simulink model "LQ_integrator_pendulum_anim"  (R2016b)
settings: Solver=ode45  StartTime=0.0  StopTime=inf  RelTol=1e-3  EnableMultiTasking=on
values from neighbouring files (symbols this model uses):
  g = 9.81    [pendulum_sys_init_solution.m]
  K_LQ = lqr(A_int,B_int,Q,R)    [pendulum_sys_init_solution.m]
  kc = 2    [pendulum_sys_init_solution.m]
  ke = 2    [pendulum_sys_init_solution.m]
  l = 1    [pendulum_sys_init_solution.m]
  M = 10    [pendulum_sys_init_solution.m]
  m = 2    [pendulum_sys_init_solution.m]
  ra = 10    [pendulum_sys_init_solution.m]
  rr = .1    (= 0.1)    [pendulum_sys_init_solution.m]
undefined symbols (not defined in the file or in its folder): pendolo_sys_diff
libraries: simulink x1, vrlib x1
settings Model: Creator=Titano  LastModifiedBy=AlessioLaBella
settings DataIOCC: LimitDataPoints=on  SaveFormat=Array  SignalLoggingSaveFormat=ModelDataLogs
settings OptimizationCC: ExpressionDepthLimit=2147483647  InitFltsAndDblsToZero=on  LifeSpan=inf
settings DebuggingCC: UnderspecifiedInitializationDetection=Classic  MergeDetectMultiDrivingBlocksExec=none  SolverPrmCheckMsg=warning  FcnCallInpInsideContextMsg=warning  StateNameClashWarn=warning  SFUnexpectedBacktrackingDiag=warning  SFNoUnconditionalDefaultTransitionDiag=warning  SFExecutionAtInitializationDiag=none
settings HardwareCC: ProdBitPerPointer=32  ProdBitPerSizeT=32  ProdBitPerPtrDiffT=32  ProdLargestAtomicFloat=None  ProdIntDivRoundTo=Undefined  ProdEndianess=Unspecified  ProdWordSize=32  ProdHWDeviceType=32-bit Generic
settings ModelReferenceCC: PropagateSignalLabelsOutOfModel=off
settings GRTTargetCC: TargetLangStandard=C89/C90 (ANSI)  GeneratePreprocessorConditionals=Disable all  CombineOutputUpdateFcns=off  GRTInterface=on
settings ConfigComp: CovMetricSettings=dw  CovHtmlReporting=on  CovSaveCumulativeToWorkspaceVar=on  CovSaveSingleToWorkspaceVar=on  CovExternalEMLEnable=off
settings SimMechanicsCC: VisDuringSimulation=on
settings ConfigurationSet: Description=SimMechanics 2G

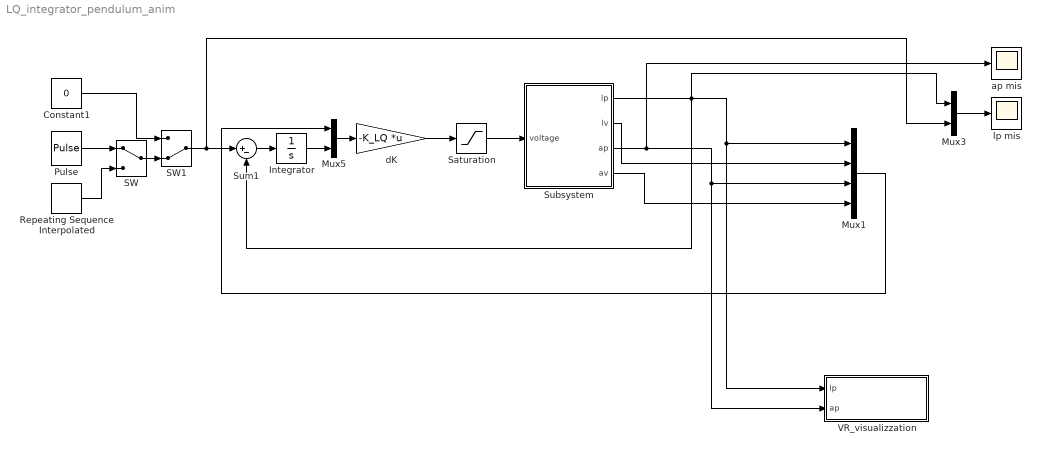
== system LQ_integrator_pendulum_anim ==
  Constant1 : Constant  Value=0
  Integrator : Integrator
  Mux1 : Mux
  Mux3 : Mux  Inputs=2
  Mux5 : Mux  Inputs=2
  Pulse : DiscretePulseGenerator  PulseType=Time based  Amplitude=.5  Period=20  PulseWidth=50
  Repeating Sequence Interpolated : simulink/Sources/Repeating Sequence Interpolated  OutValues=[.5 -.5 -.5 .5 .5].'  TimeValues=[0 2.5 5 7.5 10].'  LookUpMeth=Interpolation-Use End Values  tsamp=0.01  OutMin=[]  OutMax=[]  OutDataTypeStr=float('double')  OutputDataTypeScalingMode=Specify via dialog  OutDataType=float('double')  OutScaling=2^-10
  SW : ManualSwitch
  SW1 : ManualSwitch  CurrentSetting=0
  Saturation : Saturate  UpperLimit=24  LowerLimit=-24
  Subsystem : Subsystem
  Sum1 : Sum  Inputs=|+-
  VR_visualizzation : Subsystem
  ap mis : Scope
  dK : Gain  Gain=-K_LQ  Multiplication=Matrix(K*u)
  lp mis : Scope
  wires:
  Subsystem/3(ap) -> ap mis/1, Mux1/3, VR_visualizzation/2(ap)
  Subsystem/1(lp) -> Mux3/1, Sum1/2, VR_visualizzation/1(lp), Mux1/1
  Mux3/1 -> lp mis/1
  Constant1/1 -> SW1/1
  Mux1/1 -> Mux5/1
  SW1/1 -> Mux3/2, Sum1/1
  Sum1/1 -> Integrator/1
  Integrator/1 -> Mux5/2
  Mux5/1 -> dK/1
  SW/1 -> SW1/2
  Pulse/1 -> SW/1
  Repeating Sequence Interpolated/1 -> SW/2
  Subsystem/2(lv) -> Mux1/2
  Subsystem/4(av) -> Mux1/4
  dK/1 -> Saturation/1
  Saturation/1 -> Subsystem/1(voltage)

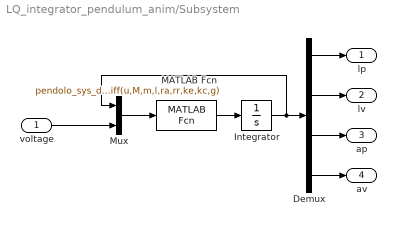
== system LQ_integrator_pendulum_anim/Subsystem ==
  voltage : Inport
  Demux : Demux
  Integrator : Integrator  InitialCondition=[0 0 0.1 0]
  MATLAB Fcn : MATLABFcn  MATLABFcn=pendolo_sys_diff(u,M,m,l,ra,rr,ke,kc,g)
  Mux : Mux  Inputs=2
  lp : Outport
  lv : Outport  Port=2
  ap : Outport  Port=3
  av : Outport  Port=4
  wires:
  MATLAB Fcn/1 -> Integrator/1
  Integrator/1 -> Demux/1, Mux/1
  Demux/4 -> av/1
  Demux/3 -> ap/1
  Demux/2 -> lv/1
  Demux/1 -> lp/1
  Mux/1 -> MATLAB Fcn/1
  voltage/1 -> Mux/2

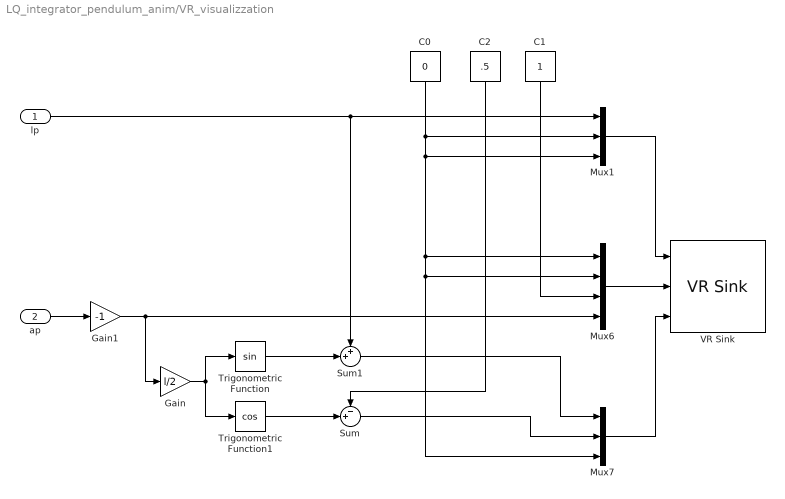
== system LQ_integrator_pendulum_anim/VR_visualizzation ==
  lp : Inport
  ap : Inport  Port=2
  C0 : Constant  Value=0
  C1 : Constant
  C2 : Constant  Value=.5
  Gain : Gain  Gain=l/2
  Gain1 : Gain  Gain=-1
  Mux1 : Mux  Inputs=3
  Mux6 : Mux
  Mux7 : Mux  Inputs=3
  Sum : Sum  Inputs=-+|
  Sum1 : Sum  Inputs=++|
  Trigonometric Function : Trigonometry
  Trigonometric Function1 : Trigonometry  Operator=cos
  VR Sink : vrlib/VR Sink  InstantiateOnLoad=on  SampleTime=0.02  ViewEnable=on  RemoteChange=off  RemoteView=off  FieldsWritten=carrello.translation.3.1.double#asta.rotation.4.1.double#asta.translation.3.1.double  WorldFileName=vrml1.wrl  AutoView=on  VideoDimensions=[]  AllowVariableSize=off  FigureProperties="{'Position', 'Name', 'Viewpoint', 'CameraBound', 'CameraDirection', 'CameraPosition', 'CameraUpVector', 'ZoomFactor', 'Antialiasing', 'Headlight', 'Lighting', 'NavPanel', 'Sound', 'StatusBar', 'Stereo3D', 'Stereo3DCameraOffset', 'Stereo3DHIT', 'ToolBar', 'Textures', 'Transparency', 'Triad', 'Wireframe', 'NavZones', 'NavMode', 'NavSpeed', 'CaptureFileFormat', 'CaptureFileName', 'Record2DCompressMethod', 'Record2DCompressQuality', 'Record2D', 'Record2DFileName', 'Record2DFPS'; [5.0000000000000000e+00   9.2333333333333371e+01   5.7600000000000000e+02   3.5000000000000000e+02], '', '', 'on', [0.0000000000000000e+00   0.0000000000000000e+00  -1.0000000000000000e+00], [0.0000000000000000e+00   0.0000000000000000e+00   1.0000000000000000e+01], [0.0000000000000000e+00   1.0000000000000000e+00   0.0000000000000000e+00], [1.0000000000000000e+00], 'on', 'on', 'on', 'halfbar', 'on', 'on', 'off', [1.0000000149011612e-01], [0.0000000000000000e+00], 'on', 'on', 'on', 'none', 'off', 'off', 'walk', 'normal', 'tif', '%f_anim_%n.tif', 'auto', [7.5000000000000000e+01], 'off', '%f_anim_%n.avi', 'auto'}"
  wires:
  Mux1/1 -> VR Sink/1
  Mux6/1 -> VR Sink/2
  Mux7/1 -> VR Sink/3
  lp/1 -> Mux1/1, Sum1/1
  C0/1 -> Mux1/2, Mux1/3, Mux6/1, Mux6/2, Mux7/3
  ap/1 -> Gain1/1
  C1/1 -> Mux6/3
  Trigonometric Function/1 -> Sum1/2
  Trigonometric Function1/1 -> Sum/2
  Sum1/1 -> Mux7/1
  Sum/1 -> Mux7/2
  C2/1 -> Sum/1
  Gain/1 -> Trigonometric Function/1, Trigonometric Function1/1
  Gain1/1 -> Mux6/4, Gain/1
